simulink model "figure_1_9"  (R2026a)
settings: Solver=ode5  FixedStep=1e-4
settings Model: Creator=yagmu  LastModifiedBy=yagmu

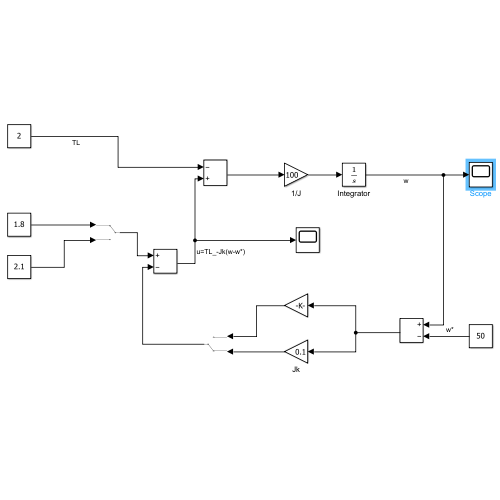
[thumbnail: Simulink's stored preview of the top-level diagram]
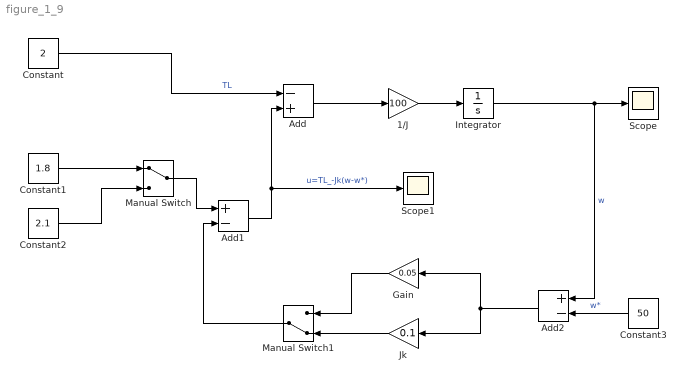
== system figure_1_9 ==
  1/J : Gain  Gain=100
  Add : Sum  Inputs=-+
  Add1 : Sum  Inputs=+-
  Add2 : Sum  Inputs=+-
  Constant : Constant  Value=2
  Constant1 : Constant  Value=1.8
  Constant2 : Constant  Value=2.1
  Constant3 : Constant  Value=50
  Gain : Gain  Gain=0.05
  Integrator : Integrator  InitialCondition=50
  Jk : Gain  Gain=0.1
  Manual Switch : ManualSwitch
  Manual Switch1 : ManualSwitch  CurrentSetting=0
  Scope : Scope
      settings: ActiveDisplayYMinimum=45.500000000007994  ActiveDisplayYMaximum=50.499999999999112
  Scope1 : Scope
  wires:
  Constant/1 -> Add/1  "TL"
  Add/1 -> 1/J/1
  1/J/1 -> Integrator/1
  Integrator/1 -> Add2/1, Scope/1  "w"
  Constant1/1 -> Manual Switch/1
  Constant2/1 -> Manual Switch/2
  Manual Switch/1 -> Add1/1
  Add1/1 -> Add/2, Scope1/1  "u=TL_-Jk(w-w*)"
  Manual Switch1/1 -> Add1/2
  Constant3/1 -> Add2/2  "w*"
  Gain/1 -> Manual Switch1/1
  Jk/1 -> Manual Switch1/2
  Add2/1 -> Jk/1, Gain/1
